simulink model "pmsm_dq_ctrl_model"  (R2020a)
settings: Solver=VariableStepAuto  StartTime=0.0  StopTime=25  RelTol=1e-3
libraries: nesl_utility x12, fl_lib x5, pmsm_dq_controller_lib x1, pmsm_dq2_lib x1
settings Model: Creator=dabagnara  LastModifiedBy=dabagnara

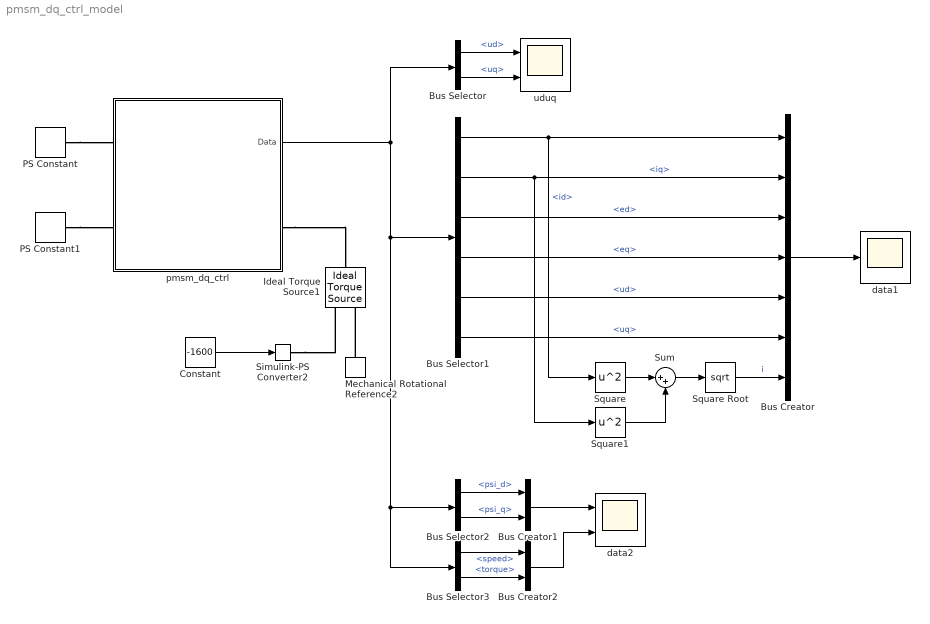
== system pmsm_dq_ctrl_model ==
  Bus Creator : BusCreator  Inputs=7
  Bus Creator1 : BusCreator  Inputs=2
  Bus Creator2 : BusCreator  Inputs=2
  Bus Selector : BusSelector  OutputSignals=ud,uq
  Bus Selector1 : BusSelector  OutputSignals=id,iq,ed,eq,ud,uq
  Bus Selector2 : BusSelector  OutputSignals=psi_d,psi_q
  Bus Selector3 : BusSelector  OutputSignals=speed,torque
  Constant : Constant  Value=-1600
  Ideal Torque Source1 : fl_lib/Mechanical/Mechanical Sources/Ideal Torque Source
  Mechanical Rotational Reference2 : fl_lib/Mechanical/Rotational Elements/Mechanical Rotational Reference
  PS Constant : fl_lib/Physical Signals/Sources/PS Constant  constant=500 rpm
  PS Constant1 : fl_lib/Physical Signals/Sources/PS Constant  constant=1750 N*m
  Simulink-PS Converter2 : nesl_utility/Simulink-PS Converter  PhysicalDomain=network_engine_domain  SubClassName=ps_input  LeftPortType=input  RightPortType=output  PseudoPeriodic=off  Frequencies=[]  NoiseDistribution=none  NoiseParameters=[]  Unit=N*m  AffineConversion=off  FilteringAndDerivatives=zero  SimscapeFilterOrder=2  InputFilterTimeConstant=0.1  UdotUserProvided=0
  Square : Math  Operator=square  SaturateOnIntegerOverflow=on
  Square Root : Sqrt  SaturateOnIntegerOverflow=on
  Square1 : Math  Operator=square  SaturateOnIntegerOverflow=on
  Sum : Sum  Inputs=|++
  data1 : Scope
  data2 : Scope  NumInputPorts=2
  pmsm_dq_ctrl : Subsystem  mask{control_mode=Speed Mode, torque_limitation=Torque limited from torque ref, ubez=616.5, ubez_unit=V, ibez=450, ibez_unit=A, omega_bez=2750, omega_bez_unit=rpm, poles=8, poles_unit=1, Rs=0.012, Rs_unit=Ohm, Ld=0.0017, Ld_unit=H, Lq=0.00429, Lq_unit=H, psi_m=0.3958 %0.5352, psi_m_unit=1, J=2.34, J_unit=kg*m^2, b=0.1, b_unit=N*m/(rad/s), kp_w=5, ki_w=20, kp_i=1, ki_i=35}
      mask prompts: control_mode "Enable Speed Mode"; torque_limitation "Enable Torque Limitation"; ubez "Nominal Voltage (phase - peak)"; ibez "Nominal Current (phase - peak)"; omega_bez "Nominal Speed"; Rs "Phase Resistance"; Ld "D-inductance"; Lq "Q-inductance"; psi_m "Magnet Flux"; J "Rotor Inertia"; b "Viscosity"; kp_w "Proportional Speed Ctrl Gain"; ki_w "Integral Speed Ctrl Gain"; kp_i "Proportional Current Ctrl Gain"; ki_i "Integral Current Ctrl Gain"
      mask init:
      | cm = get_param(gcb,'control_mode');
      | tl = get_param(gcb,'torque_limitation');
      | 
      | 
      | motor = [gcb, '/pmsm_dq2'];
      | set_param([motor],'emf_nom','ubez');
      | set_param([motor],'emf_nom_unit',ubez_unit);
      | set_param([motor],'i_nom','ibez');
      | set_param([motor],'i_nom_unit',ibez_unit);
      | set_param([motor],'omega_nom','omega_bez');
      | set_param([motor],'omega_nom_unit',omega_bez_unit);
      | set_param([motor],'poles','poles');
      | set_param([motor],'poles_unit',poles_unit);
      | set_param([motor],'Rs','Rs');
      | set_param([motor],'Rs_unit',Rs_unit);
      | set_param([motor],'Ld','Ld');
      | set_param([motor],'Ld_unit',Ld_unit);
      | set_param([motor],'Lq','Lq');
      | set_param([motor],'Lq_unit',Lq_unit);
      | set_param([motor],'psi_m','psi_m');
      | set_param([motor],'psi_m_unit',psi_m_unit);
      | set_param([motor],'J','J');
      | set_param([motor],'J_unit',J_unit);
      | set_param([motor],'b','b');
      | set_param([motor],'b_unit',b_unit);
      | 
      | controller = [gcb, '/pmsm dq controller'];
      | set_param([controller],'emf_nom','ubez');
      | set_param([controller],'emf_nom_unit',ubez_unit);
      | set_param([controller],'i_nom','ibez');
      | set_param([controller],'i_nom_unit',ibez_unit);
      | set_param([controller],'omega_m_nom','omega_bez');
      | set_param([controller],'omega_m_nom_unit',omega_bez_unit);
      | set_param([controller],'poles','poles');
      | set_param([controller],'Rs','Rs');
      | set_param([controller],'Rs_unit',Rs_unit);
      | set_param([controller],'Ld','Ld');
      | set_param([controller],'Ld_unit',Ld_unit);
      | set_param([controller],'Lq','Lq');
      | set_param([controller],'Lq_unit',Lq_unit);
      | set_param([controller],'psi_m','psi_m');
      | set_param([controller],'psi_m_unit',psi_m_unit);
      | set_param([controller],'kp_w','kp_w');
      | set_param([controller],'ki_w','ki_w');
      | set_param([controller],'kp_i','kp_i');
      | set_param([controller],'ki_i','ki_i');
      | 
      | switch cm
      |     case 'Speed Mode'
      |         set_param([controller],'Speed_mode','simscape.enum.onoff.on');
      |     case 'Torque Mode'
      |         set_param([controller],'Speed_mode','simscape.enum.onoff.off');
      | end
      | switch tl
      |     case 'Torque limited from torque ref'
      |         set_param([controller],'TorqueLim','simscape.enum.onoff.on');
      |     case 'Torque unlimited'
      |         set_param([controller],'TorqueLim','simscape.enum.onoff.off');
      | end
      mask TypeOptions control_mode: Speed Mode | Torque Mode
      mask TypeOptions torque_limitation: Torque limited from torque ref | Torque unlimited
      mask TypeOptions ubez_unit: V
      mask TypeOptions ibez_unit: A
      mask TypeOptions omega_bez_unit: rpm
      mask TypeOptions poles_unit: 1
      mask TypeOptions Rs_unit: Ohm
      mask TypeOptions Ld_unit: H
      mask TypeOptions Lq_unit: H
      mask TypeOptions psi_m_unit: 1
      mask TypeOptions J_unit: kg*m^2
      mask TypeOptions b_unit: N*m/(rad/s)
      mask DialogControl ModeofOperation Prompt: Mode of Operation
      mask DialogControl MotorParameters Prompt: Motor Parameters
      mask DialogControl ControlParameters Prompt: Control Parameters
      mask Display:
      | % Icon = 'C:\Users\dbagn\Dropbox\davide\11_matlab\11.73 HydraulicComponents\IM.jpg'
      | 
      | 
      | modelname = [gcb];
      | % image(imread("library\+pmsm_dq2\pmsm_drawing_mask.png"));
      | 
      | color('red')
      | port_label('lconn',1,'SpeedRef');
      | color('red')
      | port_label('lconn',2,'TorqueRef');
      | color('black')
      | port_label('output',1,'PMSM data');
      | color('green')
      | port_label('rconn',1,'D')
  uduq : Scope  NumInputPorts=2
  wires:
  Bus Selector/2 -> uduq/2  "<uq>"
  Bus Selector/1 -> uduq/1  "<ud>"
  Constant/1 -> Simulink-PS Converter2/1
  Bus Creator/1 -> data1/1
  Bus Selector1/1 -> Square/1, Bus Creator/1  "<id>"
  Bus Selector1/2 -> Square1/1, Bus Creator/2  "<iq>"
  Bus Selector1/3 -> Bus Creator/3  "<ed>"
  Bus Selector1/4 -> Bus Creator/4  "<eq>"
  Bus Selector1/5 -> Bus Creator/5  "<ud>"
  Bus Selector1/6 -> Bus Creator/6  "<uq>"
  Bus Creator1/1 -> data2/1
  Bus Selector2/1 -> Bus Creator1/1  "<psi_d>"
  Bus Selector2/2 -> Bus Creator1/2  "<psi_q>"
  Bus Selector3/2 -> Bus Creator2/2  "<torque>"
  Bus Selector3/1 -> Bus Creator2/1  "<speed>"
  pmsm_dq_ctrl/1(Data) -> Bus Selector3/1, Bus Selector2/1, Bus Selector1/1, Bus Selector/1
  Bus Creator2/1 -> data2/2
  Square/1 -> Sum/1
  Square1/1 -> Sum/2
  Sum/1 -> Square Root/1
  Square Root/1 -> Bus Creator/7  "i"
  connections:
  PS Constant/RConn1 -- pmsm_dq_ctrl/LConn1
  PS Constant1/RConn1 -- pmsm_dq_ctrl/LConn2
  Mechanical Rotational Reference2/LConn1 -- Ideal Torque Source1/RConn2
  Simulink-PS Converter2/RConn1 -- Ideal Torque Source1/RConn1
  pmsm_dq_ctrl/RConn1 -- Ideal Torque Source1/LConn1

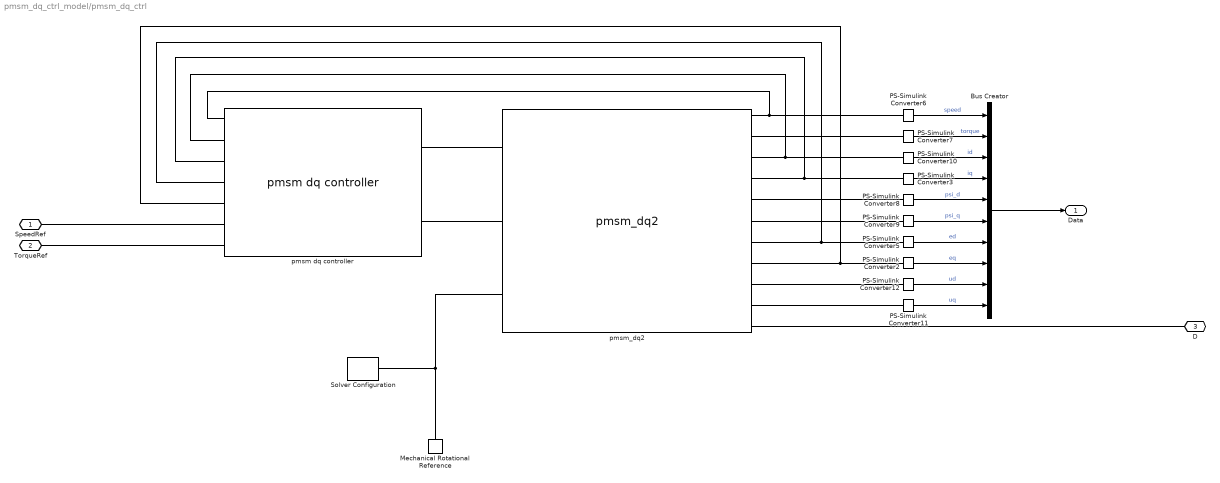
== system pmsm_dq_ctrl_model/pmsm_dq_ctrl ==
  Bus Creator : BusCreator  Inputs=10
  Mechanical Rotational Reference : fl_lib/Mechanical/Rotational Elements/Mechanical Rotational Reference
  PS-Simulink Converter10 : nesl_utility/PS-Simulink Converter  PhysicalDomain=network_engine_domain  SubClassName=ps_output  LeftPortType=input  RightPortType=output  PseudoPeriodic=off  Frequencies=[]  Unit=A  AffineConversion=on
  PS-Simulink Converter{2,5,11..12} (4 alike) : nesl_utility/PS-Simulink Converter  PhysicalDomain=network_engine_domain  SubClassName=ps_output  LeftPortType=input  RightPortType=output  PseudoPeriodic=off  Frequencies=[]  Unit=V  AffineConversion=on
  PS-Simulink Converter3 : nesl_utility/PS-Simulink Converter  PhysicalDomain=network_engine_domain  SubClassName=ps_output  LeftPortType=input  RightPortType=output  PseudoPeriodic=off  Frequencies=[]  Unit=A  AffineConversion=on
  PS-Simulink Converter6 : nesl_utility/PS-Simulink Converter  PhysicalDomain=network_engine_domain  SubClassName=ps_output  LeftPortType=input  RightPortType=output  PseudoPeriodic=off  Frequencies=[]  Unit=rpm  AffineConversion=on
  PS-Simulink Converter7 : nesl_utility/PS-Simulink Converter  PhysicalDomain=network_engine_domain  SubClassName=ps_output  LeftPortType=input  RightPortType=output  PseudoPeriodic=off  Frequencies=[]  Unit=inherit  AffineConversion=off
  PS-Simulink Converter8 : nesl_utility/PS-Simulink Converter  PhysicalDomain=network_engine_domain  SubClassName=ps_output  LeftPortType=input  RightPortType=output  PseudoPeriodic=off  Frequencies=[]  Unit=inherit  AffineConversion=off
  PS-Simulink Converter9 : nesl_utility/PS-Simulink Converter  PhysicalDomain=network_engine_domain  SubClassName=ps_output  LeftPortType=input  RightPortType=output  PseudoPeriodic=off  Frequencies=[]  Unit=inherit  AffineConversion=off
  Solver Configuration : nesl_utility/Solver Configuration  PhysicalDomain=network_engine_domain  SubClassName=solver  LeftPortType=input  RightPortType=generic  Tones=[]  Harmonics=[]  SimulateNoise=off  Profile=off  UseLocalSampling=off  EnableSwitchedLinearOptims=on  FrequencyDomain=off  UseCCode=off  RelTol=0.001  AbsTol=1e-06  MinStep=1e-09  ToWorkspace=off  RevertToSquareIcSolve=off  NumHomotopyIterations=100  PhasorMode=off  PhasorModeNumHarmonics=1  DoDC=off  ResidualTolerance=1e-09  UseLocalSolver=on  LocalSolverChoice=NE_BACKWARD_EULER_ADVANCER  LocalSolverSampleTime=tsample  DoFixedCost=on  MaxNonlinIter=3  MaxModeIter=2  LinearAlgebra=auto  EquationFormulation=NE_TIME_EF  DelaysMemoryBudget=1024  AutomaticFiltering=on  FilteringTimeConstant=tsample  PartitionStorageMethod=AS_NEEDED  PartitionMemoryBudget=1024  PartitionMethod=ROBUST
  pmsm dq controller : pmsm_dq_controller_lib/pmsm dq controller  Speed_mode=simscape.enum.onoff.on  TorqueLim=simscape.enum.onoff.on  emf_nom=ubez V  i_nom=ibez A  omega_m_nom=omega_bez rpm  poles=poles  Rs=Rs Ohm  Ld=Ld H  Lq=Lq H  psi_m=psi_m  kp_w=kp_w  ki_w=ki_w 1/s  kp_i=kp_i  ki_i=ki_i 1/s
      settings: InternalSimscapePortConfiguration="{\"Bottom\":[],\"Left\":[{\"id\":\"omega_m\",\"label\":\"__Speed__\",\"type\":\"input\"},{\"id\":\"id\",\"label\":\"_id_\",\"type\":\"input\"},{\"id\":\"iq\",\"label\":\"_iq_\",\"type\":\"input\"},{\"id\":\"ed\",\"label\":\"_ed_\",\"type\":\"input\"},{\"id\":\"eq\",\"label\":\"_eq_\",\"type\":\"input\"},{\"id\":\"omega_ref\",\"label\":\"_Speed-Set-Point_\",\"type\":\"input\"},{\"id\":\"torque_ref\",\"label\":\"_Torque-Set-Point_\",\"type\":\"input\"}],\"Right\":[{\"id\":\"ud_out\",\"label\":\"_ud_\",\"type\":\"output\"},{\"id\":\"uq_out\",\"label\":\"_uq_\",\"type\":\"output\"}],\"Top\":[]}"
  pmsm_dq2 : pmsm_dq2_lib/pmsm_dq2  emf_nom=ubez V  i_nom=ibez A  omega_nom=omega_bez rpm  poles=poles  Rs=Rs Ohm  Ld=Ld H  Lq=Lq H  psi_m=psi_m  J=J kg*m^2  b=b N*m/(rad/s)
      settings: InternalSimscapePortConfiguration="{\"Bottom\":[],\"Left\":[{\"id\":\"ud\",\"label\":\"__ud__\",\"type\":\"input\"},{\"id\":\"uq\",\"label\":\"__uq__\",\"type\":\"input\"},{\"id\":\"C\",\"label\":\"__C__\",\"type\":\"foundation.mechanical.rotational.rotational\"}],\"Right\":[{\"id\":\"omega_out\",\"label\":\"__omega_m__\",\"type\":\"output\"},{\"id\":\"tau_m\",\"label\":\"__tau_e__\",\"type\":\"output\"},{\"id\":\"id_out\",\"label\":\"__id__\",\"type\":\"output\"},{\"id\":\"iq_out\",\"label\":\"__iq__\",\"type\":\"output\"},{\"id\":\"psi_d_out\",\"label\":\"__psi_d__\",\"type\":\"output\"},{\"id\":\"psi_q_out\",\"label\":\"__psi_q__\",\"type\":\"output\"},{\"id\":\"ed_out\",\"label\":\"__ed__\",\"type\":\"output\"},{\"id\":\"eq_out\",\"label\":\"__eq__\",\"type\":\"output\"},{\"id\":\"ud_out\",\"label\":\"__ud__\",\"type\":\"output\"},{\"id\":\"uq_out\",\"label\":\"__uq__\",\"type\":\"output\"},{\"id\":\"D\",\"label\":\"__D__\",\"type\":\"foundation.mechanical.rotational.rotational\"}],\"Top\":[]}"
  SpeedRef : PMIOPort  Side=Left
  TorqueRef : PMIOPort  Port=2  Side=Left
  D : PMIOPort  Port=3  Side=Right
  Data : Outport
  wires:
  Bus Creator/1 -> Data/1
  PS-Simulink Converter8/1 -> Bus Creator/5  "psi_d"
  PS-Simulink Converter6/1 -> Bus Creator/1  "speed"
  PS-Simulink Converter7/1 -> Bus Creator/2  "torque"
  PS-Simulink Converter10/1 -> Bus Creator/3  "id"
  PS-Simulink Converter3/1 -> Bus Creator/4  "iq"
  PS-Simulink Converter9/1 -> Bus Creator/6  "psi_q"
  PS-Simulink Converter5/1 -> Bus Creator/7  "ed"
  PS-Simulink Converter2/1 -> Bus Creator/8  "eq"
  PS-Simulink Converter12/1 -> Bus Creator/9  "ud"
  PS-Simulink Converter11/1 -> Bus Creator/10  "uq"
  connections:
  PS-Simulink Converter10/LConn1 -- pmsm dq controller/LConn2 -- pmsm_dq2/RConn3
  pmsm_dq2/RConn9 -- PS-Simulink Converter12/LConn1
  pmsm_dq2/RConn10 -- PS-Simulink Converter11/LConn1
  PS-Simulink Converter3/LConn1 -- pmsm dq controller/LConn3 -- pmsm_dq2/RConn4
  pmsm_dq2/RConn6 -- PS-Simulink Converter9/LConn1
  Solver Configuration/RConn1 -- pmsm_dq2/LConn3 -- Mechanical Rotational Reference/LConn1
  PS-Simulink Converter7/LConn1 -- pmsm_dq2/RConn2
  pmsm_dq2/RConn5 -- PS-Simulink Converter8/LConn1
  pmsm dq controller/RConn1 -- pmsm_dq2/LConn1
  pmsm_dq2/RConn8 -- pmsm dq controller/LConn5 -- PS-Simulink Converter2/LConn1
  pmsm_dq2/RConn7 -- pmsm dq controller/LConn4 -- PS-Simulink Converter5/LConn1
  PS-Simulink Converter6/LConn1 -- pmsm dq controller/LConn1 -- pmsm_dq2/RConn1
  pmsm dq controller/RConn2 -- pmsm_dq2/LConn2
  pmsm_dq2/RConn11 -- D/RConn1
  TorqueRef/RConn1 -- pmsm dq controller/LConn7
  SpeedRef/RConn1 -- pmsm dq controller/LConn6
